simulink model "simulering_ROV_feedback_linearizing"  (R2020a)
settings: Solver=VariableStepAuto  StartTime=0.0  StopTime=t_sim  RelTol=1e-3
values from neighbouring files (symbols this model uses):
  D = diag([d11 d22 d33])    [constants.m]    (also in constants_dp_model.m = diag([d_11 d_22 d_33 d_44]); constants_model_coriolis.m = diag([d_11 d_22 d_33 d_44]); constants_process_model.m = diag([d_11 d_22 d_33 d_44 d_55 d_66]))
  eta0 = [x0; y0; psi0]    [constants.m]    (also in constants_dp_model.m = [x0; y0; z0; psi0]; constants_model_coriolis.m = [x0; y0; z0; psi0]; constants_process_model.m = [x0; y0; z0; phi0; theta0; psi0])
  gamma_r = 0.1    [run_simulation_FL_controller.m]    (also in run_simulation_PID_controller.m; run_simulation_SM_controller.m; run_simulation_STA_controller.m; run_simulation_feedback_linearizing.m)
  gamma_u = 0.1    [run_simulation_FL_controller.m]    (also in run_simulation_PID_controller.m; run_simulation_SM_controller.m; run_simulation_STA_controller.m; run_simulation_feedback_linearizing.m)
  gamma_v = 0.1    [run_simulation_FL_controller.m]    (also in run_simulation_PID_controller.m; run_simulation_SM_controller.m; run_simulation_STA_controller.m; run_simulation_feedback_linearizing.m)
  k_d_psi = 2*m_44*zeta_d_psi*wn_psi-d_44    [run_simulation_PID_controller.m]    (also in run_simulation_dp_model.m; run_simulation_feedback_linearizing.m = (2*1*k_p_psi*1-d33/(m_A33+m_RB33)); tuning_PID_controller.m = 2*m_66*zeta_d_psi*wn_psi-d_66; tuning_SM_controller.m = 10)
  k_d_u = (2*1*k_p_u*1-d11/(m_A11+m_RB11))    [run_simulation_feedback_linearizing.m]    (also in tuning_SM_controller.m = 5)
  k_d_v = (2*1*k_p_v*1-d22/(m_A22+m_RB22))    [run_simulation_feedback_linearizing.m]    (also in tuning_SM_controller.m = 3)
  k_i_u = k_p_u/100    (= 0.1)    [run_simulation_PID_controller.m]    (also in run_simulation_feedback_linearizing.m; tuning_PID_controller.m = k_p_u/1000)
  k_i_v = k_p_v/100    (= 0.1)    [run_simulation_PID_controller.m]    (also in run_simulation_feedback_linearizing.m; tuning_PID_controller.m = k_p_v/1000)
  k_p_psi = wn_psi^2-lambda*k_p_r    [run_simulation_FL_controller.m]    (also in run_simulation_PID_controller.m = wn_psi^2*m_44; run_simulation_SM_controller.m = 1; run_simulation_dp_model.m = wn_psi^2*m_44; run_simulation_feedback_linearizing.m = tau_r_max/deg2rad(45))
  k_p_u = m_11*pole_u-d_11    [run_simulation_FL_controller.m]    (also in run_simulation_PID_controller.m = 10; run_simulation_SM_controller.m = 1; run_simulation_dp_model.m = 1; run_simulation_feedback_linearizing.m = tau_u_max/100)
  k_p_v = m_22*pole_v-d_22    [run_simulation_FL_controller.m]    (also in run_simulation_PID_controller.m = 10; run_simulation_SM_controller.m = 1; run_simulation_dp_model.m = 1; run_simulation_feedback_linearizing.m = tau_v_max/100)
  k_psi = 10    [run_simulation_feedback_linearizing.m]
  k_r = 10    [run_simulation_feedback_linearizing.m]
  k_u = 1    [run_simulation_feedback_linearizing.m]
  k_v = 10    [run_simulation_feedback_linearizing.m]
  lambda = d_44    [run_simulation_FL_controller.m]    (also in run_simulation_PID_controller.m = 1; run_simulation_SM_controller.m = 1; run_simulation_STA_controller.m = 1; run_simulation_feedback_linearizing.m = 1)
  M_A = diag([m_A11 m_A22 m_A33])    [constants.m]    (also in constants_dp_model.m = diag([m_A11 m_A22 m_A33 m_A44]); constants_model_coriolis.m = diag([m_A11 m_A22 m_A33 m_A44]); constants_process_model.m = diag([m_A11 m_A22 m_A33 m_A44 m_A55 m_A66]))
  M_RB = diag([m_RB11 m_RB22 m_RB33])    [constants.m]    (also in constants_dp_model.m = diag([m_RB11 m_RB22 m_RB33 m_RB44]); constants_model_coriolis.m = diag([m_RB11 m_RB22 m_RB33 m_RB44]); constants_process_model.m = diag([m_RB11 m_RB22 m_RB33 m_RB44 m_RB55 m_RB66]))
  ny0 = [u0; v0; r0]    [constants.m]    (also in constants_dp_model.m = [u0; v0; w0; r0]; constants_model_coriolis.m = [u0; v0; w0; r0]; constants_process_model.m = [u0; v0; w0; p0; q0; r0])
  ny_c0 = R_z(ny0(3))'*Vc    [run_simulation_feedback_linearizing.m]
  tau_r_max = sqrt(torque_co'*torque_co)    [constants_dp_model.m]    (also in constants_model_coriolis.m; constants_process_model.m; run_simulation_feedback_linearizing.m = sqrt(torque_co'*torque_co)/(m_A33+m_RB33))
  tau_u_max = (F_max*cos(alpha1)+F_max*cos(alpha2)+F_max*cos(alpha3)+F_max*cos(alpha4))    [constants_dp_model.m]    (also in constants_model_coriolis.m; constants_process_model.m; run_simulation_feedback_linearizing.m = (F_max*cos(alpha1)+F_max*cos(alpha2)+F_max*cos(alpha3)+F_max)
  tau_v_max = (F_max*sin(alpha1)-F_max*sin(alpha2)+F_max*sin(alpha3)-F_max*sin(alpha4))    [constants_dp_model.m]    (also in constants_model_coriolis.m; constants_process_model.m; run_simulation_feedback_linearizing.m = (F_max*sin(alpha1)-F_max*sin(alpha2)+F_max*sin(alpha3)-F_max)
  theta_r_hat_init = [0; 0; 0; 0; 0]    [constants.m]
  theta_u_hat_init = [0; 0]    [constants.m]
  theta_v_hat_init = [0; 0]    [constants.m]
  Vc = sim_output.disturbance.signals.values    [run_simulation_FL_controller.m]    (also in run_simulation_PID_controller.m; run_simulation_SM_controller.m; run_simulation_dp_model.m; run_simulation_feedback_linearizing.m = [Vx; Vy; 0])
libraries: simulink x3
settings Model: Creator=kenng  LastModifiedBy=kenng

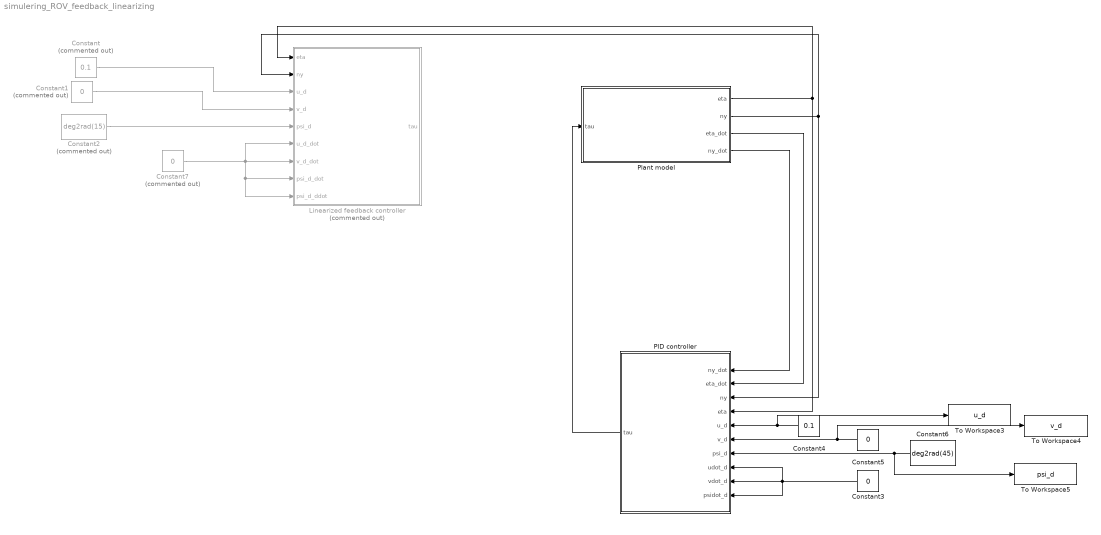
== system simulering_ROV_feedback_linearizing ==
  Constant : Constant  Commented=on  Value=0.1
  Constant1 : Constant  Commented=on  Value=0
  Constant2 : Constant  Commented=on  Value=deg2rad(15)
  Constant3 : Constant  Value=0
  Constant4 : Constant  Value=0.1
  Constant5 : Constant  Value=0
  Constant6 : Constant  Value=deg2rad(45)
  Constant7 : Constant  Commented=on  Value=0
  Linearized feedback controller : Subsystem  Commented=on
  PID controller : Subsystem
  Plant model : Subsystem
  To Workspace3 : ToWorkspace  VariableName=u_d  SaveFormat=Structure With Time  SampleTime=-1
  To Workspace4 : ToWorkspace  VariableName=v_d  SaveFormat=Structure With Time  SampleTime=-1
  To Workspace5 : ToWorkspace  VariableName=psi_d  SaveFormat=Structure With Time  SampleTime=-1
  wires:
  Constant1/1 -> Linearized feedback controller/4(v_d)
  Constant2/1 -> Linearized feedback controller/5(psi_d)
  Plant model/3(eta_dot) -> PID controller/2(eta_dot)
  Plant model/4(ny_dot) -> PID controller/1(ny_dot)
  Plant model/1(eta) -> Linearized feedback controller/1(eta), PID controller/4(eta)
  Plant model/2(ny) -> Linearized feedback controller/2(ny), PID controller/3(ny)
  Constant/1 -> Linearized feedback controller/3(u_d)
  Constant3/1 -> PID controller/10(psidot_d), PID controller/8(udot_d), PID controller/9(vdot_d)
  Constant6/1 -> To Workspace5/1, PID controller/7(psi_d)
  Constant5/1 -> To Workspace4/1, PID controller/6(v_d)
  Constant4/1 -> To Workspace3/1, PID controller/5(u_d)
  Constant7/1 -> Linearized feedback controller/8(psi_d_dot), Linearized feedback controller/9(psi_d_ddot), Linearized feedback controller/7(v_d_dot), Linearized feedback controller/6(u_d_dot)
  PID controller/1(tau) -> Plant model/1(tau)

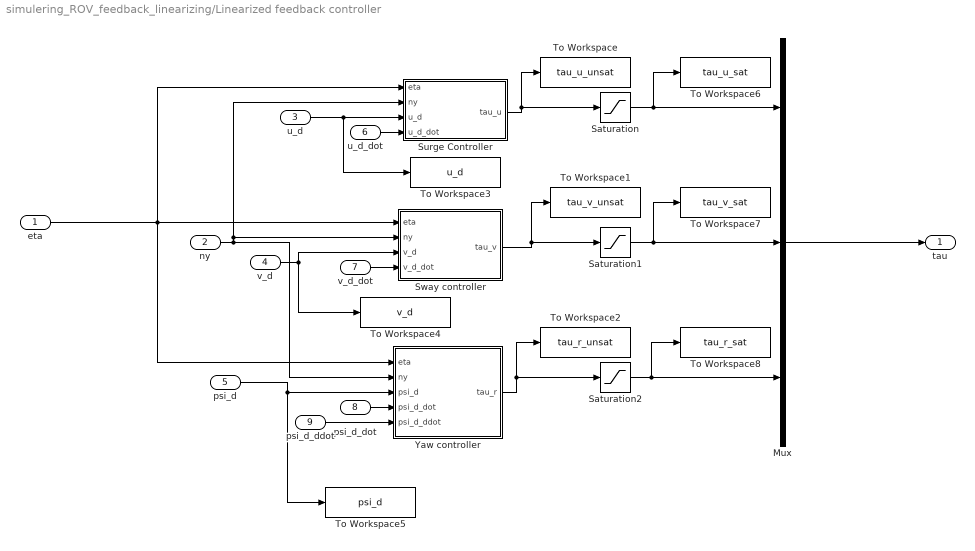
== system simulering_ROV_feedback_linearizing/Linearized feedback controller ==
  eta : Inport
  ny : Inport  Port=2
  u_d : Inport  Port=3
  v_d : Inport  Port=4
  psi_d : Inport  Port=5
  u_d_dot : Inport  Port=6
  v_d_dot : Inport  Port=7
  psi_d_dot : Inport  Port=8
  psi_d_ddot : Inport  Port=9
  Mux : Mux  Inputs=3
  Saturation : Saturate  UpperLimit=tau_u_max  LowerLimit=-tau_u_max
  Saturation1 : Saturate  UpperLimit=tau_v_max  LowerLimit=-tau_v_max
  Saturation2 : Saturate  UpperLimit=tau_r_max  LowerLimit=-tau_r_max
  Surge Controller : Subsystem
  Sway controller : Subsystem
  To Workspace : ToWorkspace  VariableName=tau_u_unsat  SaveFormat=Structure With Time  SampleTime=-1
  To Workspace1 : ToWorkspace  VariableName=tau_v_unsat  SaveFormat=Structure With Time  SampleTime=-1
  To Workspace2 : ToWorkspace  VariableName=tau_r_unsat  SaveFormat=Structure With Time  SampleTime=-1
  To Workspace3 : ToWorkspace  VariableName=u_d  SaveFormat=Structure With Time  SampleTime=-1
  To Workspace4 : ToWorkspace  VariableName=v_d  SaveFormat=Structure With Time  SampleTime=-1
  To Workspace5 : ToWorkspace  VariableName=psi_d  SaveFormat=Structure With Time  SampleTime=-1
  To Workspace6 : ToWorkspace  VariableName=tau_u_sat  SaveFormat=Structure With Time  SampleTime=-1
  To Workspace7 : ToWorkspace  VariableName=tau_v_sat  SaveFormat=Structure With Time  SampleTime=-1
  To Workspace8 : ToWorkspace  VariableName=tau_r_sat  SaveFormat=Structure With Time  SampleTime=-1
  Yaw controller : Subsystem
  tau : Outport
  wires:
  Saturation1/1 -> To Workspace7/1, Mux/2
  ny/1 -> Surge Controller/2(ny), Sway controller/2(ny), Yaw controller/2(ny)
  eta/1 -> Surge Controller/1(eta), Yaw controller/1(eta), Sway controller/1(eta)
  Surge Controller/1(tau_u) -> Saturation/1, To Workspace/1
  Saturation/1 -> Mux/1, To Workspace6/1
  u_d/1 -> To Workspace3/1, Surge Controller/3(u_d)
  Sway controller/1(tau_v) -> Saturation1/1, To Workspace1/1
  v_d/1 -> To Workspace4/1, Sway controller/3(v_d)
  Yaw controller/1(tau_r) -> Saturation2/1, To Workspace2/1
  psi_d/1 -> To Workspace5/1, Yaw controller/3(psi_d)
  Saturation2/1 -> Mux/3, To Workspace8/1
  Mux/1 -> tau/1
  u_d_dot/1 -> Surge Controller/4(u_d_dot)
  v_d_dot/1 -> Sway controller/4(v_d_dot)
  psi_d_dot/1 -> Yaw controller/4(psi_d_dot)
  psi_d_ddot/1 -> Yaw controller/5(psi_d_ddot)

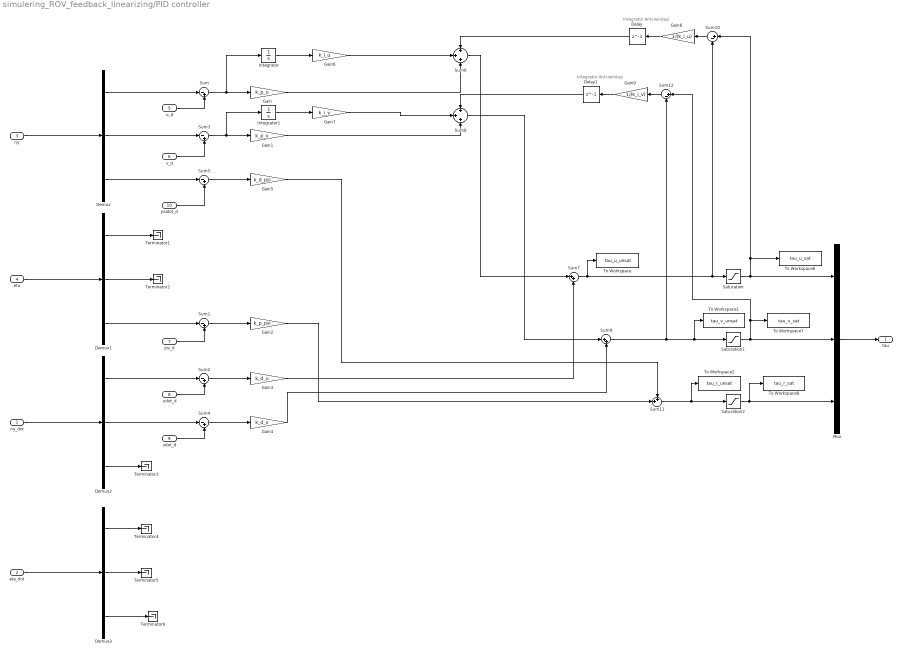
== system simulering_ROV_feedback_linearizing/PID controller ==
  note: Integrator Anti-windup
  note: Integrator Anti-windup
  ny_dot : Inport
  eta_dot : Inport  Port=2
  ny : Inport  Port=3
  eta : Inport  Port=4
  u_d : Inport  Port=5
  v_d : Inport  Port=6
  psi_d : Inport  Port=7
  udot_d : Inport  Port=8
  vdot_d : Inport  Port=9
  psidot_d : Inport  Port=10
  Delay : Delay  DelayLength=1
  Delay1 : Delay  DelayLength=1
  Demux{,1..3} (4 alike) : Demux  Outputs=3
  Gain : Gain  Gain=k_p_u
  Gain1 : Gain  Gain=k_p_v
  Gain2 : Gain  Gain=k_p_psi
  Gain3 : Gain  Gain=k_d_u
  Gain4 : Gain  Gain=k_d_v
  Gain5 : Gain  Gain=k_d_psi
  Gain6 : Gain  Gain=k_i_u
  Gain7 : Gain  Gain=k_i_v
  Gain8 : Gain  Gain=1/(k_i_u)
  Gain9 : Gain  Gain=1/(k_i_v)
  Integrator : Integrator
  Integrator1 : Integrator
  Mux : Mux  Inputs=3
  Saturation : Saturate  UpperLimit=tau_u_max  LowerLimit=-tau_u_max
  Saturation1 : Saturate  UpperLimit=tau_v_max  LowerLimit=-tau_v_max
  Saturation2 : Saturate  UpperLimit=tau_r_max  LowerLimit=-tau_r_max
  Sum{,1..5} (6 alike) : Sum  Inputs=|-+
  Sum10 : Sum  Inputs=|+-
  Sum11 : Sum  Inputs=++|
  Sum12 : Sum  Inputs=|+-
  Sum6 : Sum  Inputs=+|+|+
  Sum7 : Sum  Inputs=|++
  Sum8 : Sum  Inputs=+|+|+
  Sum9 : Sum  Inputs=|++
  Terminator{1..6} (6 alike) : Terminator
  To Workspace : ToWorkspace  VariableName=tau_u_unsat  SaveFormat=Structure With Time  SampleTime=-1
  To Workspace1 : ToWorkspace  VariableName=tau_v_unsat  SaveFormat=Structure With Time  SampleTime=-1
  To Workspace2 : ToWorkspace  VariableName=tau_r_unsat  SaveFormat=Structure With Time  SampleTime=-1
  To Workspace6 : ToWorkspace  VariableName=tau_u_sat  SaveFormat=Structure With Time  SampleTime=-1
  To Workspace7 : ToWorkspace  VariableName=tau_v_sat  SaveFormat=Structure With Time  SampleTime=-1
  To Workspace8 : ToWorkspace  VariableName=tau_r_sat  SaveFormat=Structure With Time  SampleTime=-1
  tau : Outport
  wires:
  ny/1 -> Demux/1
  Demux/3 -> Sum5/1
  Demux1/2 -> Terminator2/1
  eta/1 -> Demux1/1
  Demux1/1 -> Terminator1/1
  Demux2/3 -> Terminator3/1
  ny_dot/1 -> Demux2/1
  Demux3/2 -> Terminator5/1
  eta_dot/1 -> Demux3/1
  Demux3/1 -> Terminator4/1
  Sum/1 -> Integrator/1, Gain/1
  Sum2/1 -> Gain3/1
  Sum4/1 -> Gain4/1
  Sum5/1 -> Gain5/1
  Demux/1 -> Sum/1
  u_d/1 -> Sum/2
  v_d/1 -> Sum3/2
  Demux/2 -> Sum3/1
  Demux1/3 -> Sum1/1
  psi_d/1 -> Sum1/2
  Demux2/1 -> Sum2/1
  udot_d/1 -> Sum2/2
  Demux2/2 -> Sum4/1
  vdot_d/1 -> Sum4/2
  psidot_d/1 -> Sum5/2
  Integrator/1 -> Gain6/1
  Sum3/1 -> Integrator1/1, Gain1/1
  Integrator1/1 -> Gain7/1
  Sum1/1 -> Gain2/1
  Sum6/1 -> Sum7/1
  Gain3/1 -> Sum7/2
  Sum8/1 -> Sum9/1
  Gain4/1 -> Sum9/2
  Mux/1 -> tau/1
  Saturation2/1 -> To Workspace8/1, Mux/3
  Sum11/1 -> To Workspace2/1, Saturation2/1
  Gain2/1 -> Sum11/2
  Gain5/1 -> Sum11/1
  Sum7/1 -> Sum10/2, Saturation/1, To Workspace/1
  Sum10/1 -> Gain8/1
  Gain8/1 -> Delay/1
  Saturation/1 -> Sum10/1, To Workspace6/1, Mux/1
  Delay/1 -> Sum6/1
  Gain/1 -> Sum6/3
  Gain6/1 -> Sum6/2
  Saturation1/1 -> Sum12/1, To Workspace7/1, Mux/2
  Delay1/1 -> Sum8/1
  Sum9/1 -> Saturation1/1, To Workspace1/1, Sum12/2
  Gain9/1 -> Delay1/1
  Sum12/1 -> Gain9/1
  Gain1/1 -> Sum8/3
  Gain7/1 -> Sum8/2
  Demux3/3 -> Terminator6/1

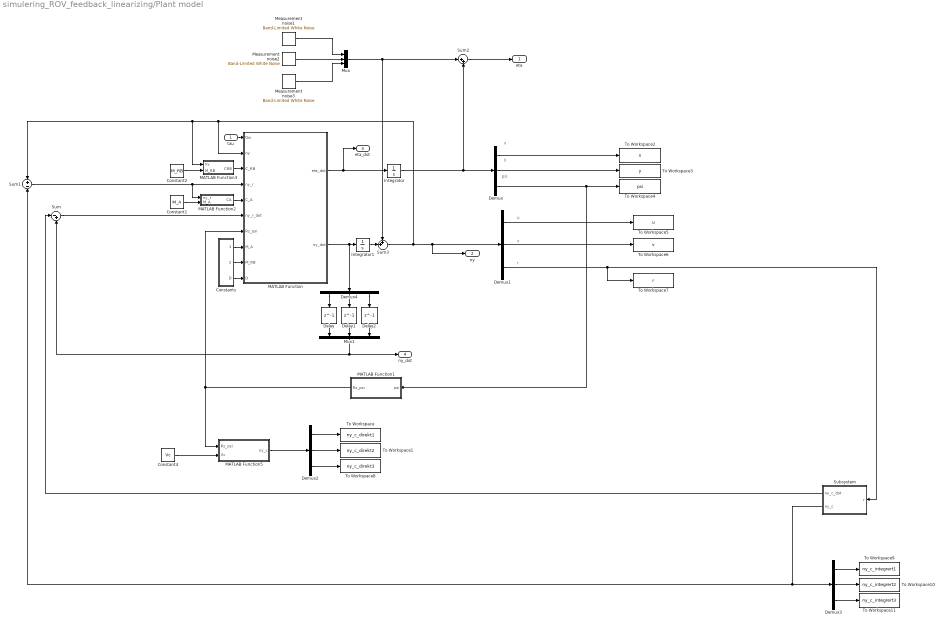
== system simulering_ROV_feedback_linearizing/Plant model ==
  note: r
  note: v
  note: u
  note: y
  note: x
  note: psi
  tau : Inport
  Constant1 : Constant  Value=M_A
  Constant2 : Constant  Value=M_RB
  Constant4 : Constant  Value=Vc
  Constants : Subsystem
  Delay : Delay  DelayLength=1
  Delay1 : Delay  DelayLength=1
  Delay2 : Delay  DelayLength=1
  Demux{,1..4} (5 alike) : Demux  Outputs=3
  Integrator : Integrator  InitialCondition=eta0
  Integrator1 : Integrator  InitialCondition=ny0
  MATLAB Function : MATLAB Function  TreatAsAtomicUnit=on
  MATLAB Function1 : MATLAB Function  TreatAsAtomicUnit=on
  MATLAB Function2 : MATLAB Function  TreatAsAtomicUnit=on
  MATLAB Function3 : MATLAB Function  TreatAsAtomicUnit=on
  MATLAB Function5 : MATLAB Function  TreatAsAtomicUnit=on
  Measurement noise1 : simulink/Sources/Band-Limited White Noise  Cov=[0.001]  Ts=.5  seed=[23341]
  Measurement noise2 : simulink/Sources/Band-Limited White Noise  Cov=[0.001]  Ts=.5  seed=[23341]
  Measurement noise3 : simulink/Sources/Band-Limited White Noise  Cov=[0.001]  Ts=.5  seed=[23341]
  Mux : Mux  Inputs=3
  Mux1 : Mux  Inputs=3
  Subsystem : Subsystem
  Sum : Sum  Inputs=|-+
  Sum1 : Sum  Inputs=+|-
  Sum2 : Sum  Inputs=|++
  Sum3 : Sum  Inputs=++|
  To Workspace : ToWorkspace  VariableName=ny_c_direkt1  SaveFormat=Structure With Time  SampleTime=-1
  To Workspace1 : ToWorkspace  VariableName=ny_c_direkt2  SaveFormat=Structure With Time  SampleTime=-1
  To Workspace10 : ToWorkspace  VariableName=ny_c_integrert2  SaveFormat=Structure With Time  SampleTime=-1
  To Workspace11 : ToWorkspace  VariableName=ny_c_integrert3  SaveFormat=Structure With Time  SampleTime=-1
  To Workspace2 : ToWorkspace  VariableName=x  SaveFormat=Structure With Time  SampleTime=-1
  To Workspace3 : ToWorkspace  VariableName=y  SaveFormat=Structure With Time  SampleTime=-1
  To Workspace4 : ToWorkspace  VariableName=psi  SaveFormat=Structure With Time  SampleTime=-1
  To Workspace5 : ToWorkspace  VariableName=u  SaveFormat=Structure With Time  SampleTime=-1
  To Workspace6 : ToWorkspace  VariableName=v  SaveFormat=Structure With Time  SampleTime=-1
  To Workspace7 : ToWorkspace  VariableName=r  SaveFormat=Structure With Time  SampleTime=-1
  To Workspace8 : ToWorkspace  VariableName=ny_c_direkt3  SaveFormat=Structure With Time  SampleTime=-1
  To Workspace9 : ToWorkspace  VariableName=ny_c_integrert1  SaveFormat=Structure With Time  SampleTime=-1
  eta : Outport
  ny : Outport  Port=2
  eta_dot : Outport  Port=3
  ny_dot : Outport  Port=4
  wires:
  Constant1/1 -> MATLAB Function2/2(M_A)
  MATLAB Function2/1(CA) -> MATLAB Function/5(C_A)
  Integrator1/1 -> Sum3/2
  MATLAB Function/1(eta_dot) -> eta_dot/1, Integrator/1
  MATLAB Function1/1(Rz_psi) -> MATLAB Function/7(Rz_psi), MATLAB Function5/1(Rz_psi)
  Integrator/1 -> Demux/1, Sum2/2
  Sum1/1 -> MATLAB Function/4(ny_r), MATLAB Function2/1(ny_r)
  Constant2/1 -> MATLAB Function3/2(M_RB)
  Subsystem/1(ny_c_dot) -> Sum/1
  tau/1 -> MATLAB Function/1(tau)
  MATLAB Function3/1(CRB) -> MATLAB Function/3(C_RB)
  Subsystem/2(ny_c) -> Demux3/1, Sum1/2
  Constant4/1 -> MATLAB Function5/2(Vc)
  Constants/1(M_A) -> MATLAB Function/8(M_A)
  Constants/2(M_RB) -> MATLAB Function/9(M_RB)
  Constants/3(D) -> MATLAB Function/10(D)
  MATLAB Function5/1(ny_c) -> Demux2/1
  Demux2/3 -> To Workspace8/1
  Demux2/1 -> To Workspace/1
  Demux2/2 -> To Workspace1/1
  Demux3/1 -> To Workspace9/1
  Demux3/2 -> To Workspace10/1
  Demux3/3 -> To Workspace11/1
  Demux/1 -> To Workspace2/1
  Demux/2 -> To Workspace3/1
  Demux/3 -> To Workspace4/1, MATLAB Function1/1(psi)
  Demux1/1 -> To Workspace5/1
  Demux1/2 -> To Workspace6/1
  Demux1/3 -> To Workspace7/1, Subsystem/1(r)
  Sum2/1 -> eta/1
  Sum3/1 -> Demux1/1, ny/1, Sum1/1, MATLAB Function3/1(ny), MATLAB Function/2(ny)
  Sum/1 -> MATLAB Function/6(ny_r_dot)
  MATLAB Function/2(ny_dot) -> Integrator1/1, Demux4/1
  Mux/1 -> Sum3/1, Sum2/1
  Measurement noise1/1 -> Mux/1
  Measurement noise2/1 -> Mux/2
  Measurement noise3/1 -> Mux/3
  Demux4/2 -> Delay1/1
  Demux4/1 -> Delay/1
  Demux4/3 -> Delay2/1
  Delay/1 -> Mux1/1
  Delay1/1 -> Mux1/2
  Delay2/1 -> Mux1/3
  Mux1/1 -> ny_dot/1, Sum/2

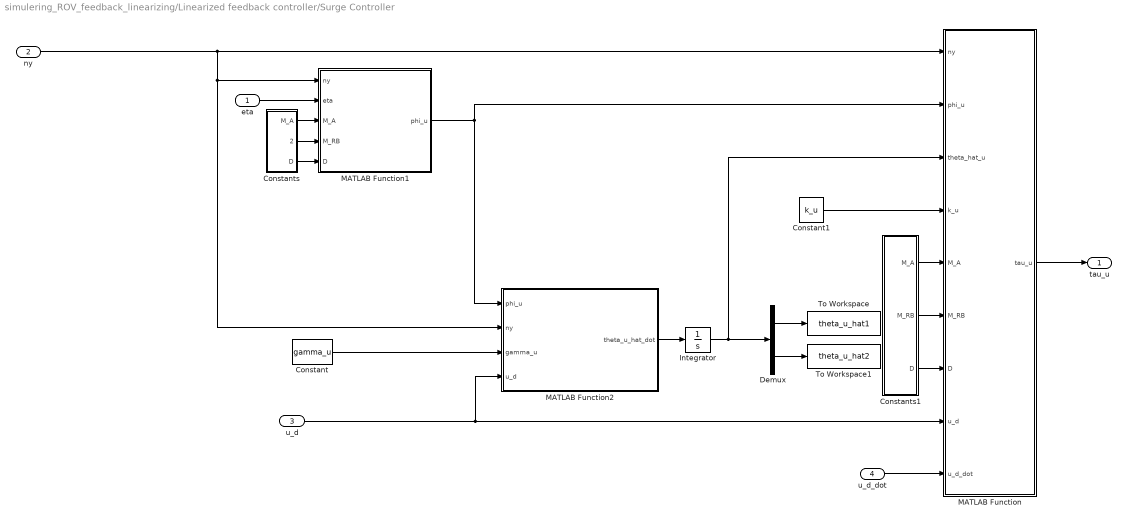
== system simulering_ROV_feedback_linearizing/Linearized feedback controller/Surge Controller ==
  eta : Inport
  ny : Inport  Port=2
  u_d : Inport  Port=3
  u_d_dot : Inport  Port=4
  Constant : Constant  Value=gamma_u
  Constant1 : Constant  Value=k_u
  Constants : Subsystem
  Constants1 : Subsystem
  Demux : Demux  Outputs=2
  Integrator : Integrator  InitialCondition=theta_u_hat_init
  MATLAB Function : MATLAB Function  TreatAsAtomicUnit=on
  MATLAB Function1 : MATLAB Function  TreatAsAtomicUnit=on
  MATLAB Function2 : MATLAB Function  TreatAsAtomicUnit=on
  To Workspace : ToWorkspace  VariableName=theta_u_hat1  SaveFormat=Structure With Time  SampleTime=-1
  To Workspace1 : ToWorkspace  VariableName=theta_u_hat2  SaveFormat=Structure With Time  SampleTime=-1
  tau_u : Outport
  wires:
  Integrator/1 -> Demux/1, MATLAB Function/3(theta_hat_u)
  MATLAB Function2/1(theta_u_hat_dot) -> Integrator/1
  MATLAB Function/1(tau_u) -> tau_u/1
  Constant1/1 -> MATLAB Function/4(k_u)
  Constant/1 -> MATLAB Function2/3(gamma_u)
  eta/1 -> MATLAB Function1/2(eta)
  u_d/1 -> MATLAB Function2/4(u_d), MATLAB Function/8(u_d)
  ny/1 -> MATLAB Function1/1(ny), MATLAB Function2/2(ny), MATLAB Function/1(ny)
  MATLAB Function1/1(phi_u) -> MATLAB Function2/1(phi_u), MATLAB Function/2(phi_u)
  Constants/1(M_A) -> MATLAB Function1/3(M_A)
  Constants/2(M_RB) -> MATLAB Function1/4(M_RB)
  Constants/3(D) -> MATLAB Function1/5(D)
  Constants1/1(M_A) -> MATLAB Function/5(M_A)
  Constants1/2(M_RB) -> MATLAB Function/6(M_RB)
  Constants1/3(D) -> MATLAB Function/7(D)
  Demux/1 -> To Workspace/1
  Demux/2 -> To Workspace1/1
  u_d_dot/1 -> MATLAB Function/9(u_d_dot)

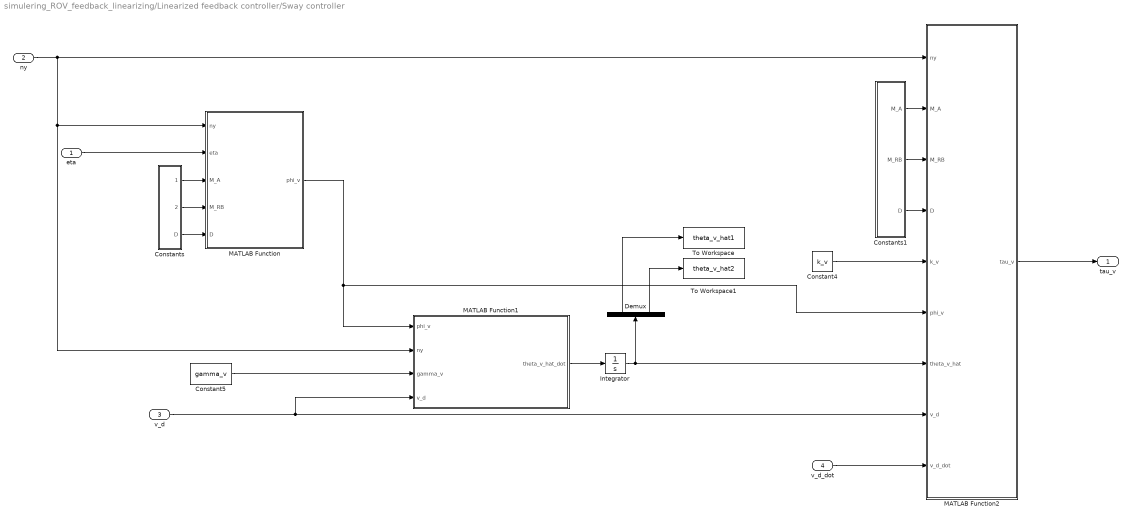
== system simulering_ROV_feedback_linearizing/Linearized feedback controller/Sway controller ==
  eta : Inport
  ny : Inport  Port=2
  v_d : Inport  Port=3
  v_d_dot : Inport  Port=4
  Constant4 : Constant  Value=k_v
  Constant5 : Constant  Value=gamma_v
  Constants : Subsystem
  Constants1 : Subsystem
  Demux : Demux  Outputs=2
  Integrator : Integrator  InitialCondition=theta_v_hat_init
  MATLAB Function : MATLAB Function  TreatAsAtomicUnit=on
  MATLAB Function1 : MATLAB Function  TreatAsAtomicUnit=on
  MATLAB Function2 : MATLAB Function  TreatAsAtomicUnit=on
  To Workspace : ToWorkspace  VariableName=theta_v_hat1  SaveFormat=Structure With Time  SampleTime=-1
  To Workspace1 : ToWorkspace  VariableName=theta_v_hat2  SaveFormat=Structure With Time  SampleTime=-1
  tau_v : Outport
  wires:
  MATLAB Function/1(phi_v) -> MATLAB Function1/1(phi_v), MATLAB Function2/6(phi_v)
  v_d/1 -> MATLAB Function2/8(v_d), MATLAB Function1/4(v_d)
  MATLAB Function1/1(theta_v_hat_dot) -> Integrator/1
  Constant4/1 -> MATLAB Function2/5(k_v)
  MATLAB Function2/1(tau_v) -> tau_v/1
  eta/1 -> MATLAB Function/2(eta)
  ny/1 -> MATLAB Function1/2(ny), MATLAB Function/1(ny), MATLAB Function2/1(ny)
  Constant5/1 -> MATLAB Function1/3(gamma_v)
  Constants/1(M_A) -> MATLAB Function/3(M_A)
  Constants/3(D) -> MATLAB Function/5(D)
  Constants/2(M_RB) -> MATLAB Function/4(M_RB)
  Constants1/1(M_A) -> MATLAB Function2/2(M_A)
  Constants1/2(M_RB) -> MATLAB Function2/3(M_RB)
  Constants1/3(D) -> MATLAB Function2/4(D)
  Demux/2 -> To Workspace1/1
  Integrator/1 -> Demux/1, MATLAB Function2/7(theta_v_hat)
  Demux/1 -> To Workspace/1
  v_d_dot/1 -> MATLAB Function2/9(v_d_dot)

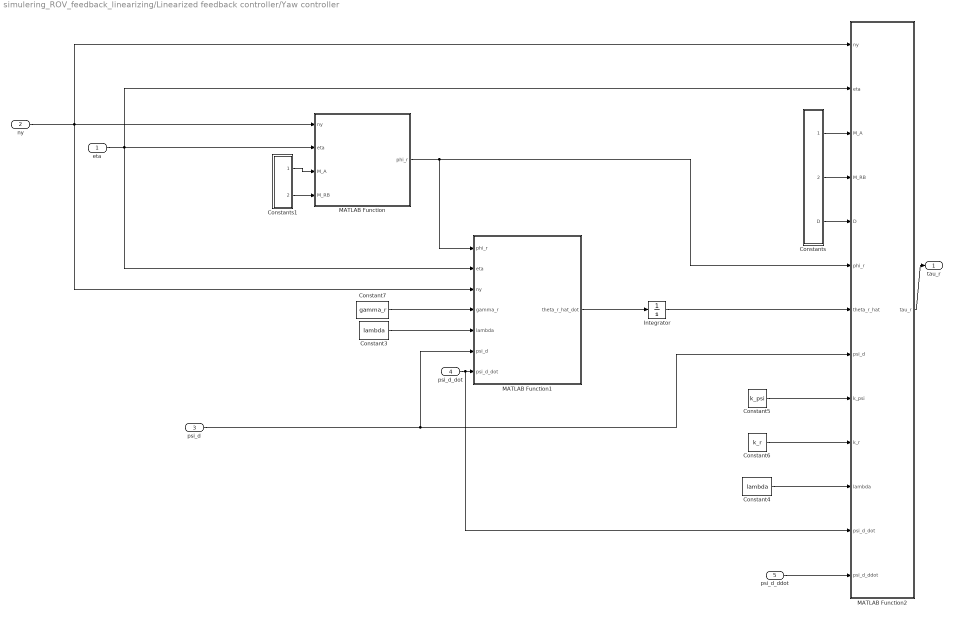
== system simulering_ROV_feedback_linearizing/Linearized feedback controller/Yaw controller ==
  eta : Inport
  ny : Inport  Port=2
  psi_d : Inport  Port=3
  psi_d_dot : Inport  Port=4
  psi_d_ddot : Inport  Port=5
  Constant3 : Constant  Value=lambda
  Constant4 : Constant  Value=lambda
  Constant5 : Constant  Value=k_psi
  Constant6 : Constant  Value=k_r
  Constant7 : Constant  Value=gamma_r
  Constants : Subsystem
  Constants1 : Subsystem
  Integrator : Integrator  InitialCondition=theta_r_hat_init
  MATLAB Function : MATLAB Function  TreatAsAtomicUnit=on
  MATLAB Function1 : MATLAB Function  TreatAsAtomicUnit=on
  MATLAB Function2 : MATLAB Function  TreatAsAtomicUnit=on
  tau_r : Outport
  wires:
  Constant4/1 -> MATLAB Function2/11(lambda)
  Constants1/2(M_RB) -> MATLAB Function/4(M_RB)
  Constant3/1 -> MATLAB Function1/5(lambda)
  MATLAB Function/1(phi_r) -> MATLAB Function2/6(phi_r), MATLAB Function1/1(phi_r)
  Integrator/1 -> MATLAB Function2/7(theta_r_hat)
  MATLAB Function1/1(theta_r_hat_dot) -> Integrator/1
  Constants/2(M_RB) -> MATLAB Function2/4(M_RB)
  Constants/1(M_A) -> MATLAB Function2/3(M_A)
  Constant7/1 -> MATLAB Function1/4(gamma_r)
  ny/1 -> MATLAB Function/1(ny), MATLAB Function2/1(ny), MATLAB Function1/3(ny)
  Constant5/1 -> MATLAB Function2/9(k_psi)
  Constants/3(D) -> MATLAB Function2/5(D)
  Constants1/1(M_A) -> MATLAB Function/3(M_A)
  Constant6/1 -> MATLAB Function2/10(k_r)
  eta/1 -> MATLAB Function1/2(eta), MATLAB Function2/2(eta), MATLAB Function/2(eta)
  MATLAB Function2/1(tau_r) -> tau_r/1
  psi_d/1 -> MATLAB Function2/8(psi_d), MATLAB Function1/6(psi_d)
  psi_d_dot/1 -> MATLAB Function2/12(psi_d_dot), MATLAB Function1/7(psi_d_dot)
  psi_d_ddot/1 -> MATLAB Function2/13(psi_d_ddot)

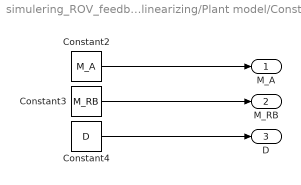
== system simulering_ROV_feedback_linearizing/Plant model/Constants ==
  Constant2 : Constant  Value=M_A
  Constant3 : Constant  Value=M_RB
  Constant4 : Constant  Value=D
  M_A : Outport
  M_RB : Outport  Port=2
  D : Outport  Port=3
  wires:
  Constant3/1 -> M_RB/1
  Constant4/1 -> D/1
  Constant2/1 -> M_A/1

== system simulering_ROV_feedback_linearizing/Plant model/Subsystem ==
  r : Inport
  Integrator : Integrator  InitialCondition=ny_c0
  MATLAB Function4 : MATLAB Function  TreatAsAtomicUnit=on
  ny_c_dot : Outport
  ny_c : Outport  Port=2
  wires:
  MATLAB Function4/1(ny_c_dot) -> Integrator/1, ny_c_dot/1
  r/1 -> MATLAB Function4/1(r)
  Integrator/1 -> MATLAB Function4/2(ny_c), ny_c/1

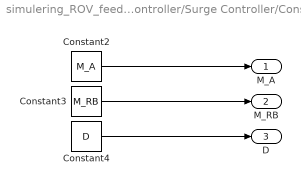
== system simulering_ROV_feedback_linearizing/Linearized feedback controller/Surge Controller/Constants ==
  Constant2 : Constant  Value=M_A
  Constant3 : Constant  Value=M_RB
  Constant4 : Constant  Value=D
  M_A : Outport
  M_RB : Outport  Port=2
  D : Outport  Port=3
  wires:
  Constant3/1 -> M_RB/1
  Constant4/1 -> D/1
  Constant2/1 -> M_A/1

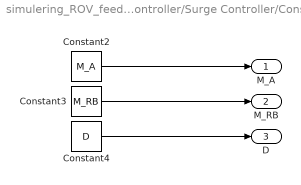
== system simulering_ROV_feedback_linearizing/Linearized feedback controller/Surge Controller/Constants1 ==
  Constant2 : Constant  Value=M_A
  Constant3 : Constant  Value=M_RB
  Constant4 : Constant  Value=D
  M_A : Outport
  M_RB : Outport  Port=2
  D : Outport  Port=3
  wires:
  Constant3/1 -> M_RB/1
  Constant4/1 -> D/1
  Constant2/1 -> M_A/1

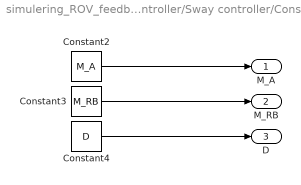
== system simulering_ROV_feedback_linearizing/Linearized feedback controller/Sway controller/Constants ==
  Constant2 : Constant  Value=M_A
  Constant3 : Constant  Value=M_RB
  Constant4 : Constant  Value=D
  M_A : Outport
  M_RB : Outport  Port=2
  D : Outport  Port=3
  wires:
  Constant3/1 -> M_RB/1
  Constant4/1 -> D/1
  Constant2/1 -> M_A/1

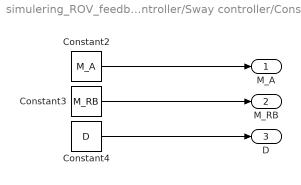
== system simulering_ROV_feedback_linearizing/Linearized feedback controller/Sway controller/Constants1 ==
  Constant2 : Constant  Value=M_A
  Constant3 : Constant  Value=M_RB
  Constant4 : Constant  Value=D
  M_A : Outport
  M_RB : Outport  Port=2
  D : Outport  Port=3
  wires:
  Constant3/1 -> M_RB/1
  Constant4/1 -> D/1
  Constant2/1 -> M_A/1

== system simulering_ROV_feedback_linearizing/Linearized feedback controller/Yaw controller/Constants ==
  Constant2 : Constant  Value=M_A
  Constant3 : Constant  Value=M_RB
  Constant4 : Constant  Value=D
  M_A : Outport
  M_RB : Outport  Port=2
  D : Outport  Port=3
  wires:
  Constant3/1 -> M_RB/1
  Constant4/1 -> D/1
  Constant2/1 -> M_A/1

== system simulering_ROV_feedback_linearizing/Linearized feedback controller/Yaw controller/Constants1 ==
  Constant2 : Constant  Value=M_A
  Constant3 : Constant  Value=M_RB
  M_A : Outport
  M_RB : Outport  Port=2
  wires:
  Constant3/1 -> M_RB/1
  Constant2/1 -> M_A/1

== matlab function simulering_ROV_feedback_linearizing/Linearized feedback controller/Surge Controller/MATLAB Function2 ==
  data: phi_u input; ny input; gamma_u input; theta_u_hat_dot output; u_d input
function theta_u_hat_dot = adaptive_law(phi_u, ny,gamma_u, u_d)
    theta_u_hat_dot = zeros(2, 1);
    theta_u_hat_dot(:, 1) = gamma_u*phi_u(:, 1)*(ny(1)-u_d);
end

== matlab function simulering_ROV_feedback_linearizing/Linearized feedback controller/Sway controller/MATLAB Function ==
  data: ny input; eta input; phi_v output; M_A input; M_RB input; D input
function phi_v = phi_v_matrix(ny, eta, M_A, M_RB, D)
    M = M_A+M_RB;
    phi_v = [-D(2,2)/M(2,2)*sin(eta(3))-(M_A(1,1)-M_A(2,2))/M(2,2)*ny(3)*cos(eta(3));
            D(2,2)/M(2,2)*cos(eta(3))-(M_A(1,1)-M_A(2,2))/M(2,2)*ny(3)*sin(eta(3))];
end

== matlab function simulering_ROV_feedback_linearizing/Linearized feedback controller/Sway controller/MATLAB Function1 ==
  data: phi_v input; ny input; gamma_v input; theta_v_hat_dot output; v_d input
function theta_v_hat_dot = adaptive_law( phi_v, ny,gamma_v, v_d)
    theta_v_hat_dot = zeros(2,1);
    theta_v_hat_dot(:, 1) = gamma_v*phi_v(:, 1)*(ny(2)-v_d);
end

== matlab function simulering_ROV_feedback_linearizing/Linearized feedback controller/Sway controller/MATLAB Function2 ==
  data: ny input; M_A input; M_RB input; tau_v output; D input; k_v input; phi_v input; theta_v_hat input; v_d input; v_d_dot input
function tau_v = sway_controller(ny, M_A, M_RB, D, k_v, phi_v, theta_v_hat, v_d, v_d_dot)
    M = M_RB+M_A;
    
    tau_v = M(1,1)/M(2,2)*ny(1)*ny(3)+D(2,2)/M(2,2)*v_d-phi_v(:,1)'*theta_v_hat(:,1)+v_d_dot-k_v*(ny(2)-v_d);

end

== matlab function simulering_ROV_feedback_linearizing/Linearized feedback controller/Yaw controller/MATLAB Function ==
  data: ny input; eta input; M_A input; phi_r output; M_RB input
function phi_r = phi_r_vec(ny, eta, M_A, M_RB)
    M = M_A + M_RB;
    phi_r = [ny(1)*sin(eta(3))-ny(2)*cos(eta(3));
            -ny(1)*cos(eta(3))-ny(2)*sin(eta(3));
            -cos(eta(3))*sin(eta(3));
            cos(eta(3))*sin(eta(3));
            1-2*sin(eta(3))*sin(eta(3))]*(M_A(1,1)-M_A(2,2))/M(3,3);
end

== matlab function simulering_ROV_feedback_linearizing/Linearized feedback controller/Yaw controller/MATLAB Function1 ==
  data: phi_r input; eta input; ny input; gamma_r input; lambda input; psi_d input; theta_r_hat_dot output; psi_d_dot input
function theta_r_hat_dot = adaptive_law(phi_r, eta, ny, gamma_r, lambda, psi_d, psi_d_dot)
    theta_r_hat_dot         = zeros(5, 1);
    theta_r_hat_dot(:,1)    = gamma_r*phi_r(:,1)*((ny(3)-psi_d_dot)+lambda*(eta(3)-psi_d));
end

== matlab function simulering_ROV_feedback_linearizing/Linearized feedback controller/Yaw controller/MATLAB Function2 ==
  data: ny input; eta input; M_A input; tau_r output; M_RB input; D input; phi_r input; theta_r_hat input; psi_d input; k_psi input; k_r input; lambda input; psi_d_dot input; psi_d_ddot input
function tau_r = yaw_controller(ny, eta, M_A, M_RB,D, phi_r, theta_r_hat,  psi_d, k_psi, k_r, lambda, psi_d_dot, psi_d_ddot)
    M = M_A + M_RB;
    tau_r = D(3,3)/M(3,3)*ny(3)-(M(1,1)-M(2,2))/M(3,3)*ny(1)*ny(2)...
        -phi_r(:,1)'*theta_r_hat(:,1)+psi_d_ddot-(k_psi+lambda*k_r)*(eta(3)-psi_d)-(k_r+lambda)*(ny(3)-psi_d_dot);
end

== matlab function simulering_ROV_feedback_linearizing/Plant model/MATLAB Function1 ==
  data: psi input; Rz_psi output
function Rz_psi = Rotation_z(psi)
Rz_psi     = [cos(psi) -sin(psi) 0;
              sin(psi) cos(psi) 0;
              0 0 1];
           
end

== matlab function simulering_ROV_feedback_linearizing/Plant model/MATLAB Function ==
  data: eta_dot output; ny_dot output; tau input; ny input; C_RB input; ny_r input; C_A input; ny_r_dot input; Rz_psi input; M_A input; M_RB input; D input
function [eta_dot, ny_dot] = vessel_system(tau, ny, C_RB, ny_r, C_A, ny_r_dot, Rz_psi, M_A, M_RB, D)
   eta_dot      = zeros(3,1);
   ny_dot       = zeros(3,1);
   eta_dot(:,1) = Rz_psi*ny(:,1);
   ny_dot(:,1) = inv(M_RB)*((M_A+M_RB)*tau(:,1)-C_RB*ny(:,1)-C_A*ny_r(:,1)-D*ny_r(:,1)-M_A*ny_r_dot(:,1));
end

== matlab function simulering_ROV_feedback_linearizing/Plant model/MATLAB Function2 ==
  data: ny_r input; M_A input; CA output
function CA = Coriolis_A(ny_r, M_A)
CA = [0 0 -M_A(2,2)*ny_r(2);
      0 0 M_A(1,1)*ny_r(1);
      M_A(2,2)*ny_r(2) -M_A(1,1)*ny_r(1) 0];
end

== matlab function simulering_ROV_feedback_linearizing/Plant model/MATLAB Function3 ==
  data: ny input; M_RB input; CRB output
function CRB = coriolis_rb(ny, M_RB)
CRB = [0 0 -M_RB(2,2)*ny(2);
       0 0 M_RB(1,1)*ny(1);
       M_RB(2,2)*ny(2) -M_RB(1,1)*ny(1) 0];
end

== matlab function simulering_ROV_feedback_linearizing/Plant model/Subsystem/MATLAB Function4 ==
  data: r input; ny_c_dot output; ny_c input
function ny_c_dot = ny_c_dynamics(r, ny_c)
ny_c_dot = [r*ny_c(2); -r*ny_c(1); 0];
end

== matlab function simulering_ROV_feedback_linearizing/Plant model/MATLAB Function5 ==
  data: ny_c output; Rz_psi input; Vc input
function ny_c = calc_nyc(Rz_psi, Vc)
ny_c = Rz_psi'*Vc;
end

== matlab function simulering_ROV_feedback_linearizing/Linearized feedback controller/Surge Controller/MATLAB Function ==
  data: ny input; phi_u input; theta_hat_u input; k_u input; M_A input; tau_u output; M_RB input; D input; u_d input; u_d_dot input
function tau_u = surge_controller(ny, phi_u, theta_hat_u, k_u, M_A, M_RB, D, u_d, u_d_dot)
    M = M_A+M_RB;
    
    tau_u = -M(2,2)/M(1,1)*ny(2)*ny(3)+D(1,1)/M(1,1)*u_d-phi_u(:,1)'*theta_hat_u(:, 1)+u_d_dot-k_u*(ny(1)-u_d);

end

== matlab function simulering_ROV_feedback_linearizing/Linearized feedback controller/Surge Controller/MATLAB Function1 ==
  data: ny input; eta input; phi_u output; M_A input; M_RB input; D input
function phi_u = phi_matrix_u(ny,eta, M_A, M_RB, D)
M = M_A + M_RB;
phi_u = [D(1,1)/M(1,1)*cos(eta(3))-(M_A(1,1)-M_A(2,2))/M(1,1)*ny(3)*sin(eta(3));
            D(1,1)/M(1,1)*sin(eta(3))+(M_A(1,1)-M_A(2,2))/M(1,1)*ny(3)*cos(eta(3))];

end
